simulink model "walkingRobotRL3D"  (R2020b)
settings: Solver=ode23t  StartTime=0.0  StopTime=Tf  RelTol=1e-2  EnableMultiTasking=on
PreLoadFcn:
  | robotParametersRL
undefined symbols (not defined in the file): agent, ankleD_pitch_jointMAX, ankleD_pitch_jointMIN, ankleD_roll_jointMAX, ankleD_roll_jointMIN, ankleI_pitch_jointMAX, ankleI_pitch_jointMIN, ankleI_roll_jointMAX, ankleI_roll_jointMIN, getSampleTime, height_plane, hipD_pitch_jointMAX, hipD_pitch_jointMIN, hipD_roll_jointMAX, hipD_roll_jointMIN, hipI_pitch_jointMAX, hipI_pitch_jointMIN, hipI_roll_jointMAX, hipI_roll_jointMIN, init_angs_L, init_angs_R, init_height, joint_damping, joint_limit_damping, joint_limit_stiffness, joint_stiffness, kneeD_jointMAX, kneeD_jointMIN, kneeI_jointMAX, kneeI_jointMIN, lower_leg_I0, lower_leg_length, lower_leg_mass, lower_leg_x, lower_leg_y, muscle_nominal_length, p10_ankleD_roll, plane_x, plane_y, regulator_type, tau, Tf, torso_height, torso_length, torso_offset_x, torso_offset_z, torso_width, torso_x, torso_y, torso_z, Ts, upper_leg_I0, upper_leg_length, upper_leg_mass, upper_leg_x, upper_leg_y, v10_ankleD_pitch, v10_ankleD_roll, v10_ankleI_pitch, v10_ankleI_roll ... (+41)
libraries: sm_lib x222, simulink x183, nesl_utility x130, walkingRobotUtils x69, rllib x2
(part 18 of 24)

== matlab function walkingRobotRL3D/Walking Robot (Angle based)/Antagonistic PAM Left Leg/kneeI PAM/Proportional Regulator (Muscles 2) ==
  data: V1 input; reg_type input; p1 output
% Author: Eduardo Reyero Ibáñez
% Descrition: In this file it will be implemented the required input for the PAM
function p1  = propReg(V1,reg_type)
%% Proportional pressure regulators VPPM
%Range of Voltage
minVoltage = 0;
maxVoltage = 7.98; % This voltage provide 8 bar of pressure with regulator type 1
p1 = zeros(1,1);
%Select regulartor type
%reg_type = 1; % This will be given by the call of the function
%Limit the voltage
for i=1:length(p1)
if V1(i) >= maxVoltage 
    V1(i) = maxVoltage;
end
end
if reg_type == 1
    f_prop = @(V) 0.99*V+0.1;
    for i=1:length(p1)
    p1(i) = f_prop(V1(i));
    end
elseif reg_type == 2
    f_prop = @(V) 0.594*V+0.06;
    for i=1:length(p1)
    p1(i) = f_prop(V1(i));
    end
else
    f_prop = @(V) 0.198*V+0.02;
    for i=1:length(p1)
    p1(i) = f_prop(V1(i));
    end
end

% figure
% fplot(p1)
% xlim([0 10])
% ylim([0 10])
end

== matlab function walkingRobotRL3D/Walking Robot (Angle based)/Antagonistic PAM Left Leg/kneeI PAM/Spring and damping model/Stimation of spring coefficients ==
  data: P1 input; S1 output; Fload input; dmax1 input; F1 input; dmax1_per input
%Author: Eduardo Reyero
%Description: Calculate spring coefficient

function S1 = calculateSpringCoeff(P1,Fload,dmax1,F1,dmax1_per)
S1=zeros(length(dmax1),1);
%curve1 = @(x,P)  -0.002697-93.8*x+2.917*P+13.05*x^2-0.04264*x*P-0.001793*P^2-0.9395*x^3-0.001597*x^2*P-0.0001142*x*P^2+4.694e-06*P^3+0.03335*x^4+6.106e-06*x^3*P+2.699e-06*x^2*P^2+1.25e-07*x*P^3-5.675e-09*P^4-0.0004611*x^5+9.334e-07*x^4*P-1.221e-08*x^3*P^2-1.463e-09*x^2*P^3-4.929e-11*x*P^4+2.492e-12*P^5;
%F1 = zeros(length(P1),1);
for i=1:length(P1)
 %   F1(i) = curve1(dmax1_per(i),P1(i)); %Should be 0 (or aprox 0)
    S1(i) = (F1(i)-Fload(i))/dmax1(i); 
end
 
 %   S1(i) = 4379.43006090932;
end

== matlab function walkingRobotRL3D/Walking Robot (Angle based)/Antagonistic PAM Left Leg/kneeI PAM/Spring and damping model/Stimation of spring coefficients1 ==
  data: F2 input; P2 input; S2 output; Fload input; dmax2 input; dmax2_per input
%Author: Eduardo Reyero
%Description: Calculate spring coefficient

function S2 = calculateSpringCoeff(F2,P2,Fload,dmax2,dmax2_per)
S2=zeros(length(dmax2),1);
%curve1 = @(x,P)  -0.002697-93.8*x+2.917*P+13.05*x^2-0.04264*x*P-0.001793*P^2-0.9395*x^3-0.001597*x^2*P-0.0001142*x*P^2+4.694e-06*P^3+0.03335*x^4+6.106e-06*x^3*P+2.699e-06*x^2*P^2+1.25e-07*x*P^3-5.675e-09*P^4-0.0004611*x^5+9.334e-07*x^4*P-1.221e-08*x^3*P^2-1.463e-09*x^2*P^3-4.929e-11*x*P^4+2.492e-12*P^5;
%F2 = zeros(length(P2),1);
for i=1:length(P2)
   % F2(i) = curve1(dmax2_per(i),P2(i)); %Should be aprox 0
    S2(i) = (F2(i)-Fload(i))/dmax2(i); 
end
  %  S2(i) = -8268.02654048148;
end

== matlab function walkingRobotRL3D/Walking Robot (Angle based)/Antagonistic PAM Left Leg/kneeI PAM/Spring and damping model/getDeltaXmax/getMaxStroke1 ==
  data: P1 input; x_max1 output
%Author: Eduardo Reyero Ibáñez
%Description: Functions for obtaining the maximun stroke value of a given
%curve F(x). It is reached for the x value which makes F = 0
function x_max1 = getMaxStroke(P1)
x_range = (-3:0.01:29)'; %This range convers the %contraction for all the pressures from 0 to 8 bar
%load('StaticFxPmodel\fxpSurface.mat');

curve1 = @(x,P)  -0.002697-93.8*x+2.917*P+13.05*x^2-0.04264*x*P-0.001793*P^2-0.9395*x^3-0.001597*x^2*P-0.0001142*x*P^2+4.694e-06*P^3+0.03335*x^4+6.106e-06*x^3*P+2.699e-06*x^2*P^2+1.25e-07*x*P^3-5.675e-09*P^4-0.0004611*x^5+9.334e-07*x^4*P-1.221e-08*x^3*P^2-1.463e-09*x^2*P^3-4.929e-11*x*P^4+2.492e-12*P^5;
F_x = zeros(length(x_range),1);
for i=1:length(x_range)
    F_x(i) = curve1(x_range(i),P1);
    if F_x(i)<0
       %We have found the x axis cross
       x_max1 = x_range(i-1);
       break;
   else
        x_max1 = x_range(i); %Will never end here but need to avoid simulink error
    end
end

end

== matlab function walkingRobotRL3D/Walking Robot (Angle based)/Antagonistic PAM Left Leg/kneeI PAM/Spring and damping model/getDeltaXmax1/getMaxStroke1 ==
  data: P2 input; x_max1 output
%Author: Eduardo Reyero Ibáñez
%Description: Functions for obtaining the maximun stroke value of a given
%curve F(x). It is reached for the x value which makes F = 0
function x_max1 = getMaxStroke(P2)
x_range = (-3:0.01:29)'; %This range convers the %contraction for all the pressures from 0 to 8 bar
%load('StaticFxPmodel\fxpSurface.mat');

curve1 = @(x,P)  -0.002697-93.8*x+2.917*P+13.05*x^2-0.04264*x*P-0.001793*P^2-0.9395*x^3-0.001597*x^2*P-0.0001142*x*P^2+4.694e-06*P^3+0.03335*x^4+6.106e-06*x^3*P+2.699e-06*x^2*P^2+1.25e-07*x*P^3-5.675e-09*P^4-0.0004611*x^5+9.334e-07*x^4*P-1.221e-08*x^3*P^2-1.463e-09*x^2*P^3-4.929e-11*x*P^4+2.492e-12*P^5;
F_x = zeros(length(x_range),1);
for i=1:length(x_range)
    F_x(i) = curve1(x_range(i),P2);
    if F_x(i)<0
       %We have found the x axis cross
       x_max1 = x_range(i-1);
       break;
   else
        x_max1 = x_range(i); %Will never end here but need to avoid simulink error
    end
end

end

== matlab function walkingRobotRL3D/Walking Robot (Angle based)/Antagonistic PAM Right Leg/Calculate Torque ==
  data: F1 input; torque output; F2 input; x1 input; x2 input; q output
%Author: Eduardo Reyero
%Description: Calculate torque based on pulley system
function [torque,q] = calculateTorque(F1,F2,x1,x2)
r_pulley = 0.03;
q = 0;
x10_ankleD_roll = 14.06*0.26/100; % In (m)
x20_ankleD_roll = 14.05*0.26/100; % In (m)
torque = (F1(1) - F2(1))*r_pulley;
q =(abs(x1(1)-x10_ankleD_roll)+abs(x2(1)-x20_ankleD_roll))/r_pulley;
if x1 >= x10_ankleD_roll
    q = q;
else
    q = - q;
end
if q > 5*pi/36
    q = 5*pi/36;
end
if q < -7*pi/36
    q = -7*pi/36;
end
end

== matlab function walkingRobotRL3D/Walking Robot1/Dynamic model of antagonistic PAM actuators/Spring//Damping (Muscles 1)/Getxmax1/getMaxStroke3 ==
  data: P1 input; x_max1 output
%Author: Eduardo Reyero Ibáñez
%Description: Functions for obtaining the maximun stroke value of a given
%curve F(x). It is reached for the x value which makes F = 0
function x_max1 = getMaxStroke(P1)
x_range = (-3:0.01:29)'; %This range convers the %contraction for all the pressures from 0 to 8 bar
%load('StaticFxPmodel\fxpSurface.mat');
curve1 = @(x,P)  -0.002697-93.8*x+2.917*P+13.05*x^2-0.04264*x*P-0.001793*P^2-0.9395*x^3-0.001597*x^2*P-0.0001142*x*P^2+4.694e-06*P^3+0.03335*x^4+6.106e-06*x^3*P+2.699e-06*x^2*P^2+1.25e-07*x*P^3-5.675e-09*P^4-0.0004611*x^5+9.334e-07*x^4*P-1.221e-08*x^3*P^2-1.463e-09*x^2*P^3-4.929e-11*x*P^4+2.492e-12*P^5;
F_x = zeros(length(x_range),1);
for i=1:length(x_range)
    F_x(i) = curve1(x_range(i),P1);
    if F_x(i)<0
       %We have found the x axis cross
       x_max1 = x_range(i-1);
       break;
   else
        x_max1 = x_range(i); %Will never end here but need to avoid simulink error
    end
end

end

== matlab function walkingRobotRL3D/Walking Robot (Angle based)/Antagonistic PAM Right Leg/Calculate Torque1 ==
  data: F1 input; torque output; F2 input; x1 input; x2 input; q output
%Author: Eduardo Reyero
%Description: Calculate torque based on pulley system
function [torque,q] = calculateTorque(F1,F2,x1,x2)
r_pulley = 0.03;
q = 0;
x10_ankleD_pitch = 14.06*0.26/100; % In (m)
x20_ankleD_pitch = 14.05*0.26/100; % In (m)
torque = (F1(1) - F2(1))*r_pulley;
q =(abs(x1(1)-x10_ankleD_pitch)+abs(x2(1)-x20_ankleD_pitch))/r_pulley;
if x1 >= x10_ankleD_pitch
    q = q;
else
    q = - q;
end
if q > pi/4
    q = pi/4;
end
if q < -pi/4
    q = -pi/4;
end
end

== matlab function walkingRobotRL3D/Walking Robot (Angle based)/Antagonistic PAM Right Leg/Calculate Torque2 ==
  data: F1 input; torque output; F2 input; x1 input; x2 input; q output
%Author: Eduardo Reyero
%Description: Calculate torque based on pulley system
function [torque,q] = calculateTorque(F1,F2,x1,x2)
r_pulley = 0.05;
q = 0;
x10_kneeD = 0.32*0.26/100; 
x20_kneeD = 28.12*0.26/100;
torque = (F1(1) - F2(1))*r_pulley;
q =(abs(x1(1)-x10_kneeD)+abs(x2(1)-x20_kneeD))/r_pulley; % Knee only moves backwards
if q > pi/2
    q = pi/2;
end
if q < 0
    q = 0;
end
end

== matlab function walkingRobotRL3D/Walking Robot (Angle based)/Antagonistic PAM Right Leg/Calculate Torque3 ==
  data: F1 input; torque output; F2 input; x1 input; x2 input; q output
%Author: Eduardo Reyero
%Description: Calculate torque based on pulley system
function [torque,q] = calculateTorque(F1,F2,x1,x2)
r_pulley = 0.05;
q = 0;
x10_hipD_roll = 14.06*0.26/100; % In (m)
x20_hipD_roll = 14.05*0.26/100; % In (m)
torque = (F1(1) - F2(1))*r_pulley;
q =(abs(x1(1)-x10_hipD_roll)+abs(x2(1)-x20_hipD_roll))/r_pulley;
if x1 >= x10_hipD_roll
    q = q;
else
    q = - q;
end
if q > pi/8
    q = pi/8;
end
if q < -pi/16
    q = -pi/16;
end
end

== matlab function walkingRobotRL3D/Walking Robot (Angle based)/Antagonistic PAM Right Leg/Calculate Torque4 ==
  data: F1 input; torque output; F2 input; x1 input; x2 input; q output
%Author: Eduardo Reyero
%Description: Calculate torque based on pulley system
function [torque,q] = calculateTorque(F1,F2,x1,x2)
r_pulley = 0.05;
q = 0;
x10_hipD_pitch = 14.06*0.26/100; % In (m)
x20_hipD_pitch = 14.05*0.26/100; % In (m)
torque = (F1(1) - F2(1))*r_pulley;
q =(abs(x1(1)-x10_hipD_pitch)+abs(x2(1)-x20_hipD_pitch))/r_pulley;
if x1 >= x10_hipD_pitch
    q = q;
else
    q = - q;
end
if q > pi/4
    q = pi/4;
end
if q < -pi/4
    q = -pi/4;
end
end

== matlab function walkingRobotRL3D/Walking Robot (Angle based)/Antagonistic PAM Left Leg/Calculate Torque ==
  data: F1 input; torque output; F2 input; x1 input; x2 input; q output
%Author: Eduardo Reyero
%Description: Calculate torque based on pulley system
function [torque,q] = calculateTorque(F1,F2,x1,x2)
r_pulley = 0.03;
q = 0;
x10_ankleI_roll = 14.06*0.26/100; % In (m)
x20_ankleI_roll = 14.05*0.26/100; % In (m)
torque = (F1(1) - F2(1))*r_pulley;
q =(abs(x1(1)-x10_ankleI_roll)+abs(x2(1)-x20_ankleI_roll))/r_pulley;
if x1 >= x10_ankleI_roll
    q = q;
else
    q = - q;
end
if q > 7*pi/36
    q = 7*pi/36;
end
if q < -5*pi/36
    q = -5*pi/36;
end
end

== matlab function walkingRobotRL3D/Walking Robot (Angle based)/Antagonistic PAM Left Leg/Calculate Torque1 ==
  data: F1 input; torque output; F2 input; x1 input; x2 input; q output
%Author: Eduardo Reyero
%Description: Calculate torque based on pulley system
function [torque,q] = calculateTorque(F1,F2,x1,x2)
r_pulley = 0.03;
q = 0;
x10_ankleI_pitch = 14.06*0.26/100; % In (m)
x20_ankleI_pitch = 14.05*0.26/100; % In (m)
torque = (F1(1) - F2(1))*r_pulley;
q =(abs(x1(1)-x10_ankleI_pitch)+abs(x2(1)-x20_ankleI_pitch))/r_pulley;
if x1 >= x10_ankleI_pitch
    q = q;
else
    q = - q;
end
if q > pi/4
    q = pi/4;
end
if q < -pi/4
    q = -pi/4;
end
end

== matlab function walkingRobotRL3D/Walking Robot1/Dynamic model of antagonistic PAM actuators/Spring//Damping (Muscles 1)/Getxmax1/getMaxStroke4 ==
  data: P1 input; x_max1 output
%Author: Eduardo Reyero Ibáñez
%Description: Functions for obtaining the maximun stroke value of a given
%curve F(x). It is reached for the x value which makes F = 0
function x_max1 = getMaxStroke(P1)
x_range = (-3:0.01:29)'; %This range convers the %contraction for all the pressures from 0 to 8 bar
%load('StaticFxPmodel\fxpSurface.mat');
curve1 = @(x,P)  -0.002697-93.8*x+2.917*P+13.05*x^2-0.04264*x*P-0.001793*P^2-0.9395*x^3-0.001597*x^2*P-0.0001142*x*P^2+4.694e-06*P^3+0.03335*x^4+6.106e-06*x^3*P+2.699e-06*x^2*P^2+1.25e-07*x*P^3-5.675e-09*P^4-0.0004611*x^5+9.334e-07*x^4*P-1.221e-08*x^3*P^2-1.463e-09*x^2*P^3-4.929e-11*x*P^4+2.492e-12*P^5;
F_x = zeros(length(x_range),1);
for i=1:length(x_range)
    F_x(i) = curve1(x_range(i),P1);
    if F_x(i)<0
       %We have found the x axis cross
       x_max1 = x_range(i-1);
       break;
   else
        x_max1 = x_range(i); %Will never end here but need to avoid simulink error
    end
end

end

== matlab function walkingRobotRL3D/Walking Robot (Angle based)/Antagonistic PAM Left Leg/Calculate Torque2 ==
  data: F1 input; torque output; F2 input; x1 input; x2 input; q output
%Author: Eduardo Reyero
%Description: Calculate torque based on pulley system
function [torque,q] = calculateTorque(F1,F2,x1,x2)
r_pulley = 0.05;
q = 0;
x10_kneeI = 0.32*0.26/100; 
x20_kneeI = 28.12*0.26/100;
torque = (F1(1) - F2(1))*r_pulley;
q =(abs(x1(1)-x10_kneeI)+abs(x2(1)-x20_kneeI))/r_pulley; % Knee only moves backwards
if q > pi/2
    q = pi/2;
end
if q < 0
    q = 0;
end
end

== matlab function walkingRobotRL3D/Walking Robot (Angle based)/Antagonistic PAM Left Leg/Calculate Torque3 ==
  data: F1 input; torque output; F2 input; x1 input; x2 input; q output
%Author: Eduardo Reyero
%Description: Calculate torque based on pulley system
function [torque,q] = calculateTorque(F1,F2,x1,x2)
r_pulley = 0.05;
q = 0;
x10_hipI_roll = 14.06*0.26/100; % In (m)
x20_hipI_roll = 14.05*0.26/100; % In (m)
torque = (F1(1) - F2(1))*r_pulley;
q =(abs(x1(1)-x10_hipI_roll)+abs(x2(1)-x20_hipI_roll))/r_pulley;
if x1 >= x10_hipI_roll
    q = q;
else
    q = - q;
end
if q > pi/16
    q = pi/16;
end
if q < -pi/8
    q = -pi/8;
end
end

== matlab function walkingRobotRL3D/Walking Robot (Angle based)/Antagonistic PAM Left Leg/Calculate Torque4 ==
  data: F1 input; torque output; F2 input; x1 input; x2 input; q output
%Author: Eduardo Reyero
%Description: Calculate torque based on pulley system
function [torque,q] = calculateTorque(F1,F2,x1,x2)
r_pulley = 0.05;
q = 0;
x10_hipI_pitch = 14.06*0.26/100; % In (m)
x20_hipI_pitch = 14.05*0.26/100; % In (m)
torque = (F1(1) - F2(1))*r_pulley;
q =(abs(x1(1)-x10_hipI_pitch)+abs(x2(1)-x20_hipI_pitch))/r_pulley;
if x1 >= x10_hipI_pitch
    q = q;
else
    q = - q;
end
if q > pi/4
    q = pi/4;
end
if q < -pi/4
    q = -pi/4;
end
end

== matlab function walkingRobotRL3D/Walking Robot (Angle based)/Dynamic model of antagonistic PAM actuators/Spring//Damping (Muscles 2)/Getxmax2/Get_delta_xmax1/getDeltaXmax4/getMaxStroke ==
  data: P2 input; x_max2 output
%Author: Eduardo Reyero Ibáñez
%Description: Functions for obtaining the maximun stroke value of a given
%curve F(x). It is reached for the x value which makes F = 0
function x_max2 = getMaxStroke(P2)
x_range = (-3:0.01:29)'; %This range convers the %contraction for all the pressures from 0 to 8 bar
%load('StaticFxPmodel\fxpSurface.mat');
curve1 = @(x,P)  -0.002697-93.8*x+2.917*P+13.05*x^2-0.04264*x*P-0.001793*P^2-0.9395*x^3-0.001597*x^2*P-0.0001142*x*P^2+4.694e-06*P^3+0.03335*x^4+6.106e-06*x^3*P+2.699e-06*x^2*P^2+1.25e-07*x*P^3-5.675e-09*P^4-0.0004611*x^5+9.334e-07*x^4*P-1.221e-08*x^3*P^2-1.463e-09*x^2*P^3-4.929e-11*x*P^4+2.492e-12*P^5;
F_x = zeros(length(x_range),1);
for i=1:length(x_range)
    F_x(i) = curve1(x_range(i),P2);
    if F_x(i)<0
       %We have found the x axis cross
       x_max2 = x_range(i-1);
       break;
   else
        x_max2 = x_range(i); %Will never end here but need to avoid simulink error
    end
end

end

== matlab function walkingRobotRL3D/Walking Robot (Angle based)/Dynamic model of antagonistic PAM actuators/Spring//Damping (Muscles 2)/Getxmax2/Get_delta_xmax1/getDeltaXmax5/MATLAB Function ==
  data: x input; savex output; xant input; save input
function savex = fcn(x,xant,save)
dif = x-xant;
if dif ~=0
    savex = xant;
else
    savex = save; %Will be the previous
end
end

== matlab function walkingRobotRL3D/Walking Robot (Angle based)/Dynamic model of antagonistic PAM actuators/Spring//Damping (Muscles 2)/Getxmax2/Get_delta_xmax1/getDeltaXmax5/getMaxStroke ==
  data: P2 input; x_max2 output
%Author: Eduardo Reyero Ibáñez
%Description: Functions for obtaining the maximun stroke value of a given
%curve F(x). It is reached for the x value which makes F = 0
function x_max2 = getMaxStroke(P2)
x_range = (-3:0.01:29)'; %This range convers the %contraction for all the pressures from 0 to 8 bar
%load('StaticFxPmodel\fxpSurface.mat');
curve1 = @(x,P)  -0.002697-93.8*x+2.917*P+13.05*x^2-0.04264*x*P-0.001793*P^2-0.9395*x^3-0.001597*x^2*P-0.0001142*x*P^2+4.694e-06*P^3+0.03335*x^4+6.106e-06*x^3*P+2.699e-06*x^2*P^2+1.25e-07*x*P^3-5.675e-09*P^4-0.0004611*x^5+9.334e-07*x^4*P-1.221e-08*x^3*P^2-1.463e-09*x^2*P^3-4.929e-11*x*P^4+2.492e-12*P^5;
F_x = zeros(length(x_range),1);
for i=1:length(x_range)
    F_x(i) = curve1(x_range(i),P2);
    if F_x(i)<0
       %We have found the x axis cross
       x_max2 = x_range(i-1);
       break;
   else
        x_max2 = x_range(i); %Will never end here but need to avoid simulink error
    end
end

end

== matlab function walkingRobotRL3D/Walking Robot (Angle based)/Dynamic model of antagonistic PAM actuators/Spring//Damping (Muscles 2)/Getxmax2/Get_delta_xmax1/getDeltaXmax6/MATLAB Function ==
  data: x input; savex output; xant input; save input
function savex = fcn(x,xant,save)
dif = x-xant;
if dif ~=0
    savex = xant;
else
    savex = save; %Will be the previous
end
end

== matlab function walkingRobotRL3D/Walking Robot (Angle based)/Dynamic model of antagonistic PAM actuators/Spring//Damping (Muscles 2)/Getxmax2/Get_delta_xmax1/getDeltaXmax6/getMaxStroke ==
  data: P2 input; x_max2 output
%Author: Eduardo Reyero Ibáñez
%Description: Functions for obtaining the maximun stroke value of a given
%curve F(x). It is reached for the x value which makes F = 0
function x_max2 = getMaxStroke(P2)
x_range = (-3:0.01:29)'; %This range convers the %contraction for all the pressures from 0 to 8 bar
%load('StaticFxPmodel\fxpSurface.mat');
curve1 = @(x,P)  -0.002697-93.8*x+2.917*P+13.05*x^2-0.04264*x*P-0.001793*P^2-0.9395*x^3-0.001597*x^2*P-0.0001142*x*P^2+4.694e-06*P^3+0.03335*x^4+6.106e-06*x^3*P+2.699e-06*x^2*P^2+1.25e-07*x*P^3-5.675e-09*P^4-0.0004611*x^5+9.334e-07*x^4*P-1.221e-08*x^3*P^2-1.463e-09*x^2*P^3-4.929e-11*x*P^4+2.492e-12*P^5;
F_x = zeros(length(x_range),1);
for i=1:length(x_range)
    F_x(i) = curve1(x_range(i),P2);
    if F_x(i)<0
       %We have found the x axis cross
       x_max2 = x_range(i-1);
       break;
   else
        x_max2 = x_range(i); %Will never end here but need to avoid simulink error
    end
end

end

== matlab function walkingRobotRL3D/Walking Robot1/Dynamic model of antagonistic PAM actuators/Spring//Damping (Muscles 1)/Getxmax1/getMaxStroke5 ==
  data: P1 input; x_max1 output
%Author: Eduardo Reyero Ibáñez
%Description: Functions for obtaining the maximun stroke value of a given
%curve F(x). It is reached for the x value which makes F = 0
function x_max1 = getMaxStroke(P1)
x_range = (-3:0.01:29)'; %This range convers the %contraction for all the pressures from 0 to 8 bar
%load('StaticFxPmodel\fxpSurface.mat');
curve1 = @(x,P)  -0.002697-93.8*x+2.917*P+13.05*x^2-0.04264*x*P-0.001793*P^2-0.9395*x^3-0.001597*x^2*P-0.0001142*x*P^2+4.694e-06*P^3+0.03335*x^4+6.106e-06*x^3*P+2.699e-06*x^2*P^2+1.25e-07*x*P^3-5.675e-09*P^4-0.0004611*x^5+9.334e-07*x^4*P-1.221e-08*x^3*P^2-1.463e-09*x^2*P^3-4.929e-11*x*P^4+2.492e-12*P^5;
F_x = zeros(length(x_range),1);
for i=1:length(x_range)
    F_x(i) = curve1(x_range(i),P1);
    if F_x(i)<0
       %We have found the x axis cross
       x_max1 = x_range(i-1);
       break;
   else
        x_max1 = x_range(i); %Will never end here but need to avoid simulink error
    end
end

end

== matlab function walkingRobotRL3D/Walking Robot (Angle based)/Dynamic model of antagonistic PAM actuators/Spring//Damping (Muscles 2)/Getxmax2/Get_delta_xmax1/getDeltaXmax7/MATLAB Function ==
  data: x input; savex output; xant input; save input
function savex = fcn(x,xant,save)
dif = x-xant;
if dif ~=0
    savex = xant;
else
    savex = save; %Will be the previous
end
end

== matlab function walkingRobotRL3D/Walking Robot (Angle based)/Dynamic model of antagonistic PAM actuators/Spring//Damping (Muscles 2)/Getxmax2/Get_delta_xmax1/getDeltaXmax7/getMaxStroke ==
  data: P2 input; x_max2 output
%Author: Eduardo Reyero Ibáñez
%Description: Functions for obtaining the maximun stroke value of a given
%curve F(x). It is reached for the x value which makes F = 0
function x_max2 = getMaxStroke(P2)
x_range = (-3:0.01:29)'; %This range convers the %contraction for all the pressures from 0 to 8 bar
%load('StaticFxPmodel\fxpSurface.mat');
curve1 = @(x,P)  -0.002697-93.8*x+2.917*P+13.05*x^2-0.04264*x*P-0.001793*P^2-0.9395*x^3-0.001597*x^2*P-0.0001142*x*P^2+4.694e-06*P^3+0.03335*x^4+6.106e-06*x^3*P+2.699e-06*x^2*P^2+1.25e-07*x*P^3-5.675e-09*P^4-0.0004611*x^5+9.334e-07*x^4*P-1.221e-08*x^3*P^2-1.463e-09*x^2*P^3-4.929e-11*x*P^4+2.492e-12*P^5;
F_x = zeros(length(x_range),1);
for i=1:length(x_range)
    F_x(i) = curve1(x_range(i),P2);
    if F_x(i)<0
       %We have found the x axis cross
       x_max2 = x_range(i-1);
       break;
   else
        x_max2 = x_range(i); %Will never end here but need to avoid simulink error
    end
end

end

== matlab function walkingRobotRL3D/Walking Robot (Angle based)/Dynamic model of antagonistic PAM actuators/Spring//Damping (Muscles 2)/Getxmax2/Get_delta_xmax1/getDeltaXmax8/MATLAB Function ==
  data: x input; savex output; xant input; save input
function savex = fcn(x,xant,save)
dif = x-xant;
if dif ~=0
    savex = xant;
else
    savex = save; %Will be the previous
end
end

== matlab function walkingRobotRL3D/Walking Robot (Angle based)/Dynamic model of antagonistic PAM actuators/Spring//Damping (Muscles 2)/Getxmax2/Get_delta_xmax1/getDeltaXmax8/getMaxStroke ==
  data: P2 input; x_max2 output
%Author: Eduardo Reyero Ibáñez
%Description: Functions for obtaining the maximun stroke value of a given
%curve F(x). It is reached for the x value which makes F = 0
function x_max2 = getMaxStroke(P2)
x_range = (-3:0.01:29)'; %This range convers the %contraction for all the pressures from 0 to 8 bar
%load('StaticFxPmodel\fxpSurface.mat');
curve1 = @(x,P)  -0.002697-93.8*x+2.917*P+13.05*x^2-0.04264*x*P-0.001793*P^2-0.9395*x^3-0.001597*x^2*P-0.0001142*x*P^2+4.694e-06*P^3+0.03335*x^4+6.106e-06*x^3*P+2.699e-06*x^2*P^2+1.25e-07*x*P^3-5.675e-09*P^4-0.0004611*x^5+9.334e-07*x^4*P-1.221e-08*x^3*P^2-1.463e-09*x^2*P^3-4.929e-11*x*P^4+2.492e-12*P^5;
F_x = zeros(length(x_range),1);
for i=1:length(x_range)
    F_x(i) = curve1(x_range(i),P2);
    if F_x(i)<0
       %We have found the x axis cross
       x_max2 = x_range(i-1);
       break;
   else
        x_max2 = x_range(i); %Will never end here but need to avoid simulink error
    end
end

end

== matlab function walkingRobotRL3D/Walking Robot (Angle based)/Dynamic model of antagonistic PAM actuators/Spring//Damping (Muscles 2)/Getxmax2/Get_delta_xmax1/getDeltaXmax9/MATLAB Function ==
  data: x input; savex output; xant input; save input
function savex = fcn(x,xant,save)
dif = x-xant;
if dif ~=0
    savex = xant;
else
    savex = save; %Will be the previous
end
end

== matlab function walkingRobotRL3D/Walking Robot (Angle based)/Dynamic model of antagonistic PAM actuators/Spring//Damping (Muscles 2)/Getxmax2/Get_delta_xmax1/getDeltaXmax9/getMaxStroke ==
  data: P2 input; x_max2 output
%Author: Eduardo Reyero Ibáñez
%Description: Functions for obtaining the maximun stroke value of a given
%curve F(x). It is reached for the x value which makes F = 0
function x_max2 = getMaxStroke(P2)
x_range = (-3:0.01:29)'; %This range convers the %contraction for all the pressures from 0 to 8 bar
%load('StaticFxPmodel\fxpSurface.mat');
curve1 = @(x,P)  -0.002697-93.8*x+2.917*P+13.05*x^2-0.04264*x*P-0.001793*P^2-0.9395*x^3-0.001597*x^2*P-0.0001142*x*P^2+4.694e-06*P^3+0.03335*x^4+6.106e-06*x^3*P+2.699e-06*x^2*P^2+1.25e-07*x*P^3-5.675e-09*P^4-0.0004611*x^5+9.334e-07*x^4*P-1.221e-08*x^3*P^2-1.463e-09*x^2*P^3-4.929e-11*x*P^4+2.492e-12*P^5;
F_x = zeros(length(x_range),1);
for i=1:length(x_range)
    F_x(i) = curve1(x_range(i),P2);
    if F_x(i)<0
       %We have found the x axis cross
       x_max2 = x_range(i-1);
       break;
   else
        x_max2 = x_range(i); %Will never end here but need to avoid simulink error
    end
end

end

== matlab function walkingRobotRL3D/Walking Robot (Angle based)/Dynamic model of antagonistic PAM actuators/Spring//Damping (Muscles 2)/MATLAB Function ==
  data: P1 input; S2 output; P2 input; delta_xmax_muscles2 input; delta_xmax_muscles1_per input; delta_xmax_muscles2_per input
%Author: Eduardo Reyero
%Description: Calculate spring coefficient

function S2 = calculateSpringCoeff2(P1,P2,delta_xmax_muscles2,delta_xmax_muscles1_per,delta_xmax_muscles2_per)
S2=zeros(length(delta_xmax_muscles2),1);
curve1 = @(x,P)  -0.002697-93.8*x+2.917*P+13.05*x^2-0.04264*x*P-0.001793*P^2-0.9395*x^3-0.001597*x^2*P-0.0001142*x*P^2+4.694e-06*P^3+0.03335*x^4+6.106e-06*x^3*P+2.699e-06*x^2*P^2+1.25e-07*x*P^3-5.675e-09*P^4-0.0004611*x^5+9.334e-07*x^4*P-1.221e-08*x^3*P^2-1.463e-09*x^2*P^3-4.929e-11*x*P^4+2.492e-12*P^5;
F1 = zeros(length(P1),1);
F2 = zeros(length(P1),1);
for i = 1:length(P2)
   F1(i) = curve1(delta_xmax_muscles1_per(i),P1(i));
   F2(i) = curve1(delta_xmax_muscles2_per(i),P2(i));
  S2(i) = (F2(i)-F1(i))/delta_xmax_muscles2(i);
  %S2(i) = F2(i)-F1(i)/(delta_xmax_muscles2_per(i)*0.26/100);
  
%    if S2(i)> 1e+05 || S2(i)< -1e+05
%        S2(i) = 0.1;
%    end
%    if S2(i)<0
%    S2(i) = -S2(i); 
%    end
end

end

== matlab function walkingRobotRL3D/Action+CI1/MATLAB Function ==
  data: x1 input; v1 output; v2 output
function [v1,v2]=ankleD_action(x1)
v1_values = [1.6809 1.72]';
v2_values = [1.6807 1.64]';
v1 = v1_values(1);
v2 = v2_values(1);
if  x1(1)>=14.05 
    v1 = v1_values(2);
    v2 = v2_values(2);
end
  
end

== matlab function walkingRobotRL3D/Walking Robot33/DYNAMIC MODEL OF PAM FOR LEFT LEG/Dynamic Model Antagonisitic PAM1/F(x,P) mode (Muscles 1) ==
  data: P1 input; F1 output; x_muscle1 input
%Author: Eduardo Reyero Ibáñez
%Note: F(x) curves for different pressures are limited by recommended
%limitation of 20% in contraction percentage for the used PAM actuator
%(L = 260mm D=20mm)
function F1 = FxPmodel(P1,x_muscle1)
%Input: P comming from proporcional controller  is in bar. Its 6x1 vector
% x_muscle (in % contraction)
%Output:F according to P input and and x value of half of the maximun
%permissible stroke
%Importing 2 variable F(x,P) model
curve = @(x,P)  -0.002697-93.8*x+2.917*P+13.05*x^2-0.04264*x*P-0.001793*P^2-0.9395*x^3-0.001597*x^2*P-0.0001142*x*P^2+4.694e-06*P^3+0.03335*x^4+6.106e-06*x^3*P+2.699e-06*x^2*P^2+1.25e-07*x*P^3-5.675e-09*P^4-0.0004611*x^5+9.334e-07*x^4*P-1.221e-08*x^3*P^2-1.463e-09*x^2*P^3-4.929e-11*x*P^4+2.492e-12*P^5;
%Defining F and x vectors for the 6 actuators
F1 = zeros(length(P1),1); %6x1
x1 = zeros(length(P1),1); %6x1
% Transform P from bar to Kpa
P1 = 100*P1;

for i=1:length(P1)
% Obtaining the stroke
x1(i) = x_muscle1(i); 
% Obtaining the applied force
F1(i) = curve(x1(i),P1(i)); 
if F1(i)<0
    F1(i) = 0;
end
end
end

== matlab function walkingRobotRL3D/Walking Robot1/Dynamic model of antagonistic PAM actuators/Spring//Damping (Muscles 2)/Getxmax2/getMaxStroke7 ==
  data: P2 input; x_max2 output
%Author: Eduardo Reyero Ibáñez
%Description: Functions for obtaining the maximun stroke value of a given
%curve F(x). It is reached for the x value which makes F = 0
function x_max2 = getMaxStroke(P2)
x_range = (-3:0.01:29)'; %This range convers the %contraction for all the pressures from 0 to 8 bar
%load('StaticFxPmodel\fxpSurface.mat');
curve1 = @(x,P)  -0.002697-93.8*x+2.917*P+13.05*x^2-0.04264*x*P-0.001793*P^2-0.9395*x^3-0.001597*x^2*P-0.0001142*x*P^2+4.694e-06*P^3+0.03335*x^4+6.106e-06*x^3*P+2.699e-06*x^2*P^2+1.25e-07*x*P^3-5.675e-09*P^4-0.0004611*x^5+9.334e-07*x^4*P-1.221e-08*x^3*P^2-1.463e-09*x^2*P^3-4.929e-11*x*P^4+2.492e-12*P^5;
F_x = zeros(length(x_range),1);
for i=1:length(x_range)
    F_x(i) = curve1(x_range(i),P2);
    if F_x(i)<0
       %We have found the x axis cross
       x_max2 = x_range(i-1);
       break;
   else
        x_max2 = x_range(i); %Will never end here but need to avoid simulink error
    end
end

end

== matlab function walkingRobotRL3D/Walking Robot33/DYNAMIC MODEL OF PAM FOR LEFT LEG/Dynamic Model Antagonisitic PAM1/F(x,P) mode (Muscles 1)1 ==
  data: P2 input; F2 output; x_muscle2 input
%Author: Eduardo Reyero Ibáñez
%Note: F(x) curves for different pressures are limited by recommended
%limitation of 20% in contraction percentage for the used PAM actuator
%(L = 260mm D=20mm)
function F2 = FxPmodel(P2,x_muscle2)
%Input: P comming from proporcional controller  is in bar. Its 6x1 vector
% x_muscle (in % contraction)
%Output:F according to P input and and x value of half of the maximun
%permissible stroke
%Importing 2 variable F(x,P) model
curve = @(x,P)  -0.002697-93.8*x+2.917*P+13.05*x^2-0.04264*x*P-0.001793*P^2-0.9395*x^3-0.001597*x^2*P-0.0001142*x*P^2+4.694e-06*P^3+0.03335*x^4+6.106e-06*x^3*P+2.699e-06*x^2*P^2+1.25e-07*x*P^3-5.675e-09*P^4-0.0004611*x^5+9.334e-07*x^4*P-1.221e-08*x^3*P^2-1.463e-09*x^2*P^3-4.929e-11*x*P^4+2.492e-12*P^5;
%Defining F and x vectors for the 6 actuators
F2 = zeros(length(P2),1); %6x1
x2 = zeros(length(P2),1); %6x1
% Transform P from bar to Kpa
P2 = 100*P2;

for i=1:length(P2)
% Obtaining the stroke
x2(i) = x_muscle2(i); 
% Obtaining the applied force
F2(i) = curve(x2(i),P2(i));
if F2(i)<0
    F2(i) = 0;
end
end
end

== matlab function walkingRobotRL3D/Walking Robot33/DYNAMIC MODEL OF PAM FOR LEFT LEG/Dynamic Model Antagonisitic PAM1/Proportional Regulator (Muscles 1) ==
  data: V1 input; reg_type input; p1 output
% Author: Eduardo Reyero Ibáñez
% Descrition: In this file it will be implemented the required input for the PAM
function p1  = propReg(V1,reg_type)
%% Proportional pressure regulators VPPM
%Range of Voltage
minVoltage = 0;
maxVoltage = 7.98; % This voltage provide 8 bar of pressure with regulator type 1
p1 = zeros(1,1);
%Select regulartor type
%reg_type = 1; % This will be given by the call of the function
%Limit the voltage
for i=1:length(p1)
if V1(i) >= maxVoltage 
    V1(i) = maxVoltage;
end
end
if reg_type == 1
    f_prop = @(V) 0.99*V+0.1;
    for i=1:length(p1)
    p1(i) = f_prop(V1(i));
    end
elseif reg_type == 2
    f_prop = @(V) 0.594*V+0.06;
    for i=1:length(p1)
    p1(i) = f_prop(V1(i));
    end
else
    f_prop = @(V) 0.198*V+0.02;
    for i=1:length(p1)
    p1(i) = f_prop(V1(i));
    end
end

% figure
% fplot(p1)
% xlim([0 10])
% ylim([0 10])
end

== matlab function walkingRobotRL3D/Walking Robot33/DYNAMIC MODEL OF PAM FOR LEFT LEG/Dynamic Model Antagonisitic PAM1/Proportional Regulator (Muscles 2) ==
  data: V1 input; reg_type input; p1 output
% Author: Eduardo Reyero Ibáñez
% Descrition: In this file it will be implemented the required input for the PAM
function p1  = propReg(V1,reg_type)
%% Proportional pressure regulators VPPM
%Range of Voltage
minVoltage = 0;
maxVoltage = 7.98; % This voltage provide 8 bar of pressure with regulator type 1
p1 = zeros(1,1);
%Select regulartor type
%reg_type = 1; % This will be given by the call of the function
%Limit the voltage
for i=1:length(p1)
if V1(i) >= maxVoltage 
    V1(i) = maxVoltage;
end
end
if reg_type == 1
    f_prop = @(V) 0.99*V+0.1;
    for i=1:length(p1)
    p1(i) = f_prop(V1(i));
    end
elseif reg_type == 2
    f_prop = @(V) 0.594*V+0.06;
    for i=1:length(p1)
    p1(i) = f_prop(V1(i));
    end
else
    f_prop = @(V) 0.198*V+0.02;
    for i=1:length(p1)
    p1(i) = f_prop(V1(i));
    end
end

% figure
% fplot(p1)
% xlim([0 10])
% ylim([0 10])
end

== matlab function walkingRobotRL3D/Walking Robot33/DYNAMIC MODEL OF PAM FOR LEFT LEG/Dynamic Model Antagonisitic PAM1/Spring and damping model/S(P),D(P) ==
  data: P1 input; S1 output; P2 input; D1 output; S2 output; D2 output
function [S1,D1,S2,D2] = getSpringDampingCoeff(P1,P2)
tau = 0.6;
% Spring and damping coeff for muscle 1
if P1>=0 && P1<=1
    S1 = 400;
    D1 = tau*S1;
elseif P1>1 && P1<=2
    S1 = 500;
    D1 = tau*S1;
elseif P1>2 && P1<=3
    S1 = 1100;
    D1 = tau*S1;
elseif P1>3 && P1<=4
    S1 = 1500;
    D1 = tau*S1;
elseif P1>4 && P1<=5
    S1 = 2000;
    D1 = tau*S1;
elseif P1>5 && P1<=6
    S1 = 2900;
    D1 = tau*S1;
elseif P1>6 && P1<=7
    S1 = 3800;
    D1 = tau*S1;
elseif P1>7 && P1<=8.5
    S1 = 5000;
    D1 = tau*S1;
else %Never will enter here
    S1 = 800;
    D1 = tau*S1;  
end

% Spring and damping coeff for muscle 1
if P2>=0 && P2<=1
    S2 = 400;
    D2 = tau*S2;
elseif P2>1 && P2<=2
    S2 = 500;
    D2 = tau*S2;
elseif P2>2 && P2<=3
    S2 = 1100;
    D2 = tau*S2;
elseif P2>3 && P2<=4
    S2 = 1500;
    D2 = tau*S2;
elseif P2>4 && P2<=5
    S2 = 2000;
    D2 = tau*S2;
elseif P2>5 && P2<=6
    S2 = 2900;
    D2 = tau*S2;
elseif P2>6 && P2<=7
    S2 = 3800;
    D2 = tau*S2;
elseif P2>7 && P2<=8.5
    S2 = 5000;
    D2 = tau*S2;
else %Never will enter here
    S2 = 800;
    D2 = tau*S2;  
end

end

== matlab function walkingRobotRL3D/Walking Robot33/DYNAMIC MODEL OF PAM FOR LEFT LEG/Dynamic Model Antagonisitic PAM2/F(x,P) mode (Muscles 1) ==
  data: P1 input; F1 output; x_muscle1 input
%Author: Eduardo Reyero Ibáñez
%Note: F(x) curves for different pressures are limited by recommended
%limitation of 20% in contraction percentage for the used PAM actuator
%(L = 260mm D=20mm)
function F1 = FxPmodel(P1,x_muscle1)
%Input: P comming from proporcional controller  is in bar. Its 6x1 vector
% x_muscle (in % contraction)
%Output:F according to P input and and x value of half of the maximun
%permissible stroke
%Importing 2 variable F(x,P) model
curve = @(x,P)  -0.002697-93.8*x+2.917*P+13.05*x^2-0.04264*x*P-0.001793*P^2-0.9395*x^3-0.001597*x^2*P-0.0001142*x*P^2+4.694e-06*P^3+0.03335*x^4+6.106e-06*x^3*P+2.699e-06*x^2*P^2+1.25e-07*x*P^3-5.675e-09*P^4-0.0004611*x^5+9.334e-07*x^4*P-1.221e-08*x^3*P^2-1.463e-09*x^2*P^3-4.929e-11*x*P^4+2.492e-12*P^5;
%Defining F and x vectors for the 6 actuators
F1 = zeros(length(P1),1); %6x1
x1 = zeros(length(P1),1); %6x1
% Transform P from bar to Kpa
P1 = 100*P1;

for i=1:length(P1)
% Obtaining the stroke
x1(i) = x_muscle1(i); 
% Obtaining the applied force
F1(i) = curve(x1(i),P1(i)); 
if F1(i)<0
    F1(i) = 0;
end
end
end

== matlab function walkingRobotRL3D/Walking Robot33/DYNAMIC MODEL OF PAM FOR LEFT LEG/Dynamic Model Antagonisitic PAM2/F(x,P) mode (Muscles 1)1 ==
  data: P2 input; F2 output; x_muscle2 input
%Author: Eduardo Reyero Ibáñez
%Note: F(x) curves for different pressures are limited by recommended
%limitation of 20% in contraction percentage for the used PAM actuator
%(L = 260mm D=20mm)
function F2 = FxPmodel(P2,x_muscle2)
%Input: P comming from proporcional controller  is in bar. Its 6x1 vector
% x_muscle (in % contraction)
%Output:F according to P input and and x value of half of the maximun
%permissible stroke
%Importing 2 variable F(x,P) model
curve = @(x,P)  -0.002697-93.8*x+2.917*P+13.05*x^2-0.04264*x*P-0.001793*P^2-0.9395*x^3-0.001597*x^2*P-0.0001142*x*P^2+4.694e-06*P^3+0.03335*x^4+6.106e-06*x^3*P+2.699e-06*x^2*P^2+1.25e-07*x*P^3-5.675e-09*P^4-0.0004611*x^5+9.334e-07*x^4*P-1.221e-08*x^3*P^2-1.463e-09*x^2*P^3-4.929e-11*x*P^4+2.492e-12*P^5;
%Defining F and x vectors for the 6 actuators
F2 = zeros(length(P2),1); %6x1
x2 = zeros(length(P2),1); %6x1
% Transform P from bar to Kpa
P2 = 100*P2;

for i=1:length(P2)
% Obtaining the stroke
x2(i) = x_muscle2(i); 
% Obtaining the applied force
F2(i) = curve(x2(i),P2(i));
if F2(i)<0
    F2(i) = 0;
end
end
end

== matlab function walkingRobotRL3D/Walking Robot33/DYNAMIC MODEL OF PAM FOR LEFT LEG/Dynamic Model Antagonisitic PAM2/Proportional Regulator (Muscles 1) ==
  data: V1 input; reg_type input; p1 output
% Author: Eduardo Reyero Ibáñez
% Descrition: In this file it will be implemented the required input for the PAM
function p1  = propReg(V1,reg_type)
%% Proportional pressure regulators VPPM
%Range of Voltage
minVoltage = 0;
maxVoltage = 7.98; % This voltage provide 8 bar of pressure with regulator type 1
p1 = zeros(1,1);
%Select regulartor type
%reg_type = 1; % This will be given by the call of the function
%Limit the voltage
for i=1:length(p1)
if V1(i) >= maxVoltage 
    V1(i) = maxVoltage;
end
end
if reg_type == 1
    f_prop = @(V) 0.99*V+0.1;
    for i=1:length(p1)
    p1(i) = f_prop(V1(i));
    end
elseif reg_type == 2
    f_prop = @(V) 0.594*V+0.06;
    for i=1:length(p1)
    p1(i) = f_prop(V1(i));
    end
else
    f_prop = @(V) 0.198*V+0.02;
    for i=1:length(p1)
    p1(i) = f_prop(V1(i));
    end
end

% figure
% fplot(p1)
% xlim([0 10])
% ylim([0 10])
end

== matlab function walkingRobotRL3D/Walking Robot33/DYNAMIC MODEL OF PAM FOR LEFT LEG/Dynamic Model Antagonisitic PAM2/Proportional Regulator (Muscles 2) ==
  data: V1 input; reg_type input; p1 output
% Author: Eduardo Reyero Ibáñez
% Descrition: In this file it will be implemented the required input for the PAM
function p1  = propReg(V1,reg_type)
%% Proportional pressure regulators VPPM
%Range of Voltage
minVoltage = 0;
maxVoltage = 7.98; % This voltage provide 8 bar of pressure with regulator type 1
p1 = zeros(1,1);
%Select regulartor type
%reg_type = 1; % This will be given by the call of the function
%Limit the voltage
for i=1:length(p1)
if V1(i) >= maxVoltage 
    V1(i) = maxVoltage;
end
end
if reg_type == 1
    f_prop = @(V) 0.99*V+0.1;
    for i=1:length(p1)
    p1(i) = f_prop(V1(i));
    end
elseif reg_type == 2
    f_prop = @(V) 0.594*V+0.06;
    for i=1:length(p1)
    p1(i) = f_prop(V1(i));
    end
else
    f_prop = @(V) 0.198*V+0.02;
    for i=1:length(p1)
    p1(i) = f_prop(V1(i));
    end
end

% figure
% fplot(p1)
% xlim([0 10])
% ylim([0 10])
end

== matlab function walkingRobotRL3D/Walking Robot1/Dynamic model of antagonistic PAM actuators/Spring//Damping (Muscles 2)/Getxmax2/getMaxStroke ==
  data: P2 input; x_max2 output
%Author: Eduardo Reyero Ibáñez
%Description: Functions for obtaining the maximun stroke value of a given
%curve F(x). It is reached for the x value which makes F = 0
function x_max2 = getMaxStroke(P2)
x_range = (-3:0.01:29)'; %This range convers the %contraction for all the pressures from 0 to 8 bar
%load('StaticFxPmodel\fxpSurface.mat');
curve1 = @(x,P)  -0.002697-93.8*x+2.917*P+13.05*x^2-0.04264*x*P-0.001793*P^2-0.9395*x^3-0.001597*x^2*P-0.0001142*x*P^2+4.694e-06*P^3+0.03335*x^4+6.106e-06*x^3*P+2.699e-06*x^2*P^2+1.25e-07*x*P^3-5.675e-09*P^4-0.0004611*x^5+9.334e-07*x^4*P-1.221e-08*x^3*P^2-1.463e-09*x^2*P^3-4.929e-11*x*P^4+2.492e-12*P^5;
F_x = zeros(length(x_range),1);
for i=1:length(x_range)
    F_x(i) = curve1(x_range(i),P2);
    if F_x(i)<0
       %We have found the x axis cross
       x_max2 = x_range(i-1);
       break;
   else
        x_max2 = x_range(i); %Will never end here but need to avoid simulink error
    end
end

end

== matlab function walkingRobotRL3D/Action+CI33/MATLAB Function ==
  data: x1 input; v1 output; v2 output
function [v1,v2]=ankleD_action(x1)
v1_values = [1.6809 1.72]';
v2_values = [1.6807 1.64]';
v1 = v1_values(1);
v2 = v2_values(1);
if  x1(1)>=14.05 
    v1 = v1_values(2);
    v2 = v2_values(2);
end
  
end

== matlab function walkingRobotRL3D/mapActions33 ==
  data: value input; output output
function output = mapfun(value)
%narginchk(20,20)
%nargoutchk(0,20)
fromLow = -1;
fromHigh= 1;
toLow= 1.4;
toHigh= 3;
output = (value - fromLow) .* (toHigh - toLow) ./ (fromHigh - fromLow) + toLow;
end

== matlab function walkingRobotRL3D/Walking Robot/DYNAMIC MODEL OF PAM FOR LEFT LEG/Dynamic Model Antagonisitic PAM1/F(x,P) mode (Muscles 1) ==
  data: P1 input; F1 output; x_muscle1 input
%Author: Eduardo Reyero Ibáñez
%Note: F(x) curves for different pressures are limited by recommended
%limitation of 20% in contraction percentage for the used PAM actuator
%(L = 260mm D=20mm)
function F1 = FxPmodel(P1,x_muscle1)
%Input: P comming from proporcional controller  is in bar. Its 6x1 vector
% x_muscle (in % contraction)
%Output:F according to P input and and x value of half of the maximun
%permissible stroke
%Importing 2 variable F(x,P) model
curve = @(x,P)  -0.002697-93.8*x+2.917*P+13.05*x^2-0.04264*x*P-0.001793*P^2-0.9395*x^3-0.001597*x^2*P-0.0001142*x*P^2+4.694e-06*P^3+0.03335*x^4+6.106e-06*x^3*P+2.699e-06*x^2*P^2+1.25e-07*x*P^3-5.675e-09*P^4-0.0004611*x^5+9.334e-07*x^4*P-1.221e-08*x^3*P^2-1.463e-09*x^2*P^3-4.929e-11*x*P^4+2.492e-12*P^5;
%Defining F and x vectors for the 6 actuators
F1 = zeros(length(P1),1); %6x1
x1 = zeros(length(P1),1); %6x1
% Transform P from bar to Kpa
P1 = 100*P1;

for i=1:length(P1)
% Obtaining the stroke
x1(i) = x_muscle1(i); 
% Obtaining the applied force
F1(i) = curve(x1(i),P1(i)); 
if F1(i)<0
    F1(i) = 0;
end
end
end

== matlab function walkingRobotRL3D/Walking Robot/DYNAMIC MODEL OF PAM FOR LEFT LEG/Dynamic Model Antagonisitic PAM1/F(x,P) mode (Muscles 1)1 ==
  data: P2 input; F2 output; x_muscle2 input
%Author: Eduardo Reyero Ibáñez
%Note: F(x) curves for different pressures are limited by recommended
%limitation of 20% in contraction percentage for the used PAM actuator
%(L = 260mm D=20mm)
function F2 = FxPmodel(P2,x_muscle2)
%Input: P comming from proporcional controller  is in bar. Its 6x1 vector
% x_muscle (in % contraction)
%Output:F according to P input and and x value of half of the maximun
%permissible stroke
%Importing 2 variable F(x,P) model
curve = @(x,P)  -0.002697-93.8*x+2.917*P+13.05*x^2-0.04264*x*P-0.001793*P^2-0.9395*x^3-0.001597*x^2*P-0.0001142*x*P^2+4.694e-06*P^3+0.03335*x^4+6.106e-06*x^3*P+2.699e-06*x^2*P^2+1.25e-07*x*P^3-5.675e-09*P^4-0.0004611*x^5+9.334e-07*x^4*P-1.221e-08*x^3*P^2-1.463e-09*x^2*P^3-4.929e-11*x*P^4+2.492e-12*P^5;
%Defining F and x vectors for the 6 actuators
F2 = zeros(length(P2),1); %6x1
x2 = zeros(length(P2),1); %6x1
% Transform P from bar to Kpa
P2 = 100*P2;

for i=1:length(P2)
% Obtaining the stroke
x2(i) = x_muscle2(i); 
% Obtaining the applied force
F2(i) = curve(x2(i),P2(i));
if F2(i)<0
    F2(i) = 0;
end
end
end

== matlab function walkingRobotRL3D/Walking Robot/DYNAMIC MODEL OF PAM FOR LEFT LEG/Dynamic Model Antagonisitic PAM1/Proportional Regulator (Muscles 1) ==
  data: V1 input; reg_type input; p1 output
% Author: Eduardo Reyero Ibáñez
% Descrition: In this file it will be implemented the required input for the PAM
function p1  = propReg(V1,reg_type)
%% Proportional pressure regulators VPPM
%Range of Voltage
minVoltage = 0;
maxVoltage = 7.98; % This voltage provide 8 bar of pressure with regulator type 1
p1 = zeros(1,1);
%Select regulartor type
%reg_type = 1; % This will be given by the call of the function
%Limit the voltage
for i=1:length(p1)
if V1(i) >= maxVoltage 
    V1(i) = maxVoltage;
end
end
if reg_type == 1
    f_prop = @(V) 0.99*V+0.1;
    for i=1:length(p1)
    p1(i) = f_prop(V1(i));
    end
elseif reg_type == 2
    f_prop = @(V) 0.594*V+0.06;
    for i=1:length(p1)
    p1(i) = f_prop(V1(i));
    end
else
    f_prop = @(V) 0.198*V+0.02;
    for i=1:length(p1)
    p1(i) = f_prop(V1(i));
    end
end

% figure
% fplot(p1)
% xlim([0 10])
% ylim([0 10])
end

== matlab function walkingRobotRL3D/Walking Robot/DYNAMIC MODEL OF PAM FOR LEFT LEG/Dynamic Model Antagonisitic PAM1/Proportional Regulator (Muscles 2) ==
  data: V1 input; reg_type input; p1 output
% Author: Eduardo Reyero Ibáñez
% Descrition: In this file it will be implemented the required input for the PAM
function p1  = propReg(V1,reg_type)
%% Proportional pressure regulators VPPM
%Range of Voltage
minVoltage = 0;
maxVoltage = 7.98; % This voltage provide 8 bar of pressure with regulator type 1
p1 = zeros(1,1);
%Select regulartor type
%reg_type = 1; % This will be given by the call of the function
%Limit the voltage
for i=1:length(p1)
if V1(i) >= maxVoltage 
    V1(i) = maxVoltage;
end
end
if reg_type == 1
    f_prop = @(V) 0.99*V+0.1;
    for i=1:length(p1)
    p1(i) = f_prop(V1(i));
    end
elseif reg_type == 2
    f_prop = @(V) 0.594*V+0.06;
    for i=1:length(p1)
    p1(i) = f_prop(V1(i));
    end
else
    f_prop = @(V) 0.198*V+0.02;
    for i=1:length(p1)
    p1(i) = f_prop(V1(i));
    end
end

% figure
% fplot(p1)
% xlim([0 10])
% ylim([0 10])
end

== matlab function walkingRobotRL3D/Walking Robot/DYNAMIC MODEL OF PAM FOR LEFT LEG/Dynamic Model Antagonisitic PAM1/Spring and damping model/S(P),D(P) ==
  data: P1 input; S1 output; P2 input; D1 output; S2 output; D2 output
function [S1,D1,S2,D2] = getSpringDampingCoeff(P1,P2)
tau = 0.6;
% Spring and damping coeff for muscle 1
if P1>=0 && P1<=1
    S1 = 400;
    D1 = tau*S1;
elseif P1>1 && P1<=2
    S1 = 500;
    D1 = tau*S1;
elseif P1>2 && P1<=3
    S1 = 1100;
    D1 = tau*S1;
elseif P1>3 && P1<=4
    S1 = 1500;
    D1 = tau*S1;
elseif P1>4 && P1<=5
    S1 = 2000;
    D1 = tau*S1;
elseif P1>5 && P1<=6
    S1 = 2900;
    D1 = tau*S1;
elseif P1>6 && P1<=7
    S1 = 3800;
    D1 = tau*S1;
elseif P1>7 && P1<=8.5
    S1 = 5000;
    D1 = tau*S1;
else %Never will enter here
    S1 = 800;
    D1 = tau*S1;  
end

% Spring and damping coeff for muscle 1
if P2>=0 && P2<=1
    S2 = 400;
    D2 = tau*S2;
elseif P2>1 && P2<=2
    S2 = 500;
    D2 = tau*S2;
elseif P2>2 && P2<=3
    S2 = 1100;
    D2 = tau*S2;
elseif P2>3 && P2<=4
    S2 = 1500;
    D2 = tau*S2;
elseif P2>4 && P2<=5
    S2 = 2000;
    D2 = tau*S2;
elseif P2>5 && P2<=6
    S2 = 2900;
    D2 = tau*S2;
elseif P2>6 && P2<=7
    S2 = 3800;
    D2 = tau*S2;
elseif P2>7 && P2<=8.5
    S2 = 5000;
    D2 = tau*S2;
else %Never will enter here
    S2 = 800;
    D2 = tau*S2;  
end

end

== matlab function walkingRobotRL3D/Walking Robot/DYNAMIC MODEL OF PAM FOR LEFT LEG/Dynamic Model Antagonisitic PAM2/F(x,P) mode (Muscles 1) ==
  data: P1 input; F1 output; x_muscle1 input
%Author: Eduardo Reyero Ibáñez
%Note: F(x) curves for different pressures are limited by recommended
%limitation of 20% in contraction percentage for the used PAM actuator
%(L = 260mm D=20mm)
function F1 = FxPmodel(P1,x_muscle1)
%Input: P comming from proporcional controller  is in bar. Its 6x1 vector
% x_muscle (in % contraction)
%Output:F according to P input and and x value of half of the maximun
%permissible stroke
%Importing 2 variable F(x,P) model
curve = @(x,P)  -0.002697-93.8*x+2.917*P+13.05*x^2-0.04264*x*P-0.001793*P^2-0.9395*x^3-0.001597*x^2*P-0.0001142*x*P^2+4.694e-06*P^3+0.03335*x^4+6.106e-06*x^3*P+2.699e-06*x^2*P^2+1.25e-07*x*P^3-5.675e-09*P^4-0.0004611*x^5+9.334e-07*x^4*P-1.221e-08*x^3*P^2-1.463e-09*x^2*P^3-4.929e-11*x*P^4+2.492e-12*P^5;
%Defining F and x vectors for the 6 actuators
F1 = zeros(length(P1),1); %6x1
x1 = zeros(length(P1),1); %6x1
% Transform P from bar to Kpa
P1 = 100*P1;

for i=1:length(P1)
% Obtaining the stroke
x1(i) = x_muscle1(i); 
% Obtaining the applied force
F1(i) = curve(x1(i),P1(i)); 
if F1(i)<0
    F1(i) = 0;
end
end
end

== matlab function walkingRobotRL3D/Walking Robot1/Dynamic model of antagonistic PAM actuators/Spring//Damping (Muscles 2)/Getxmax2/getMaxStroke1 ==
  data: P2 input; x_max2 output
%Author: Eduardo Reyero Ibáñez
%Description: Functions for obtaining the maximun stroke value of a given
%curve F(x). It is reached for the x value which makes F = 0
function x_max2 = getMaxStroke(P2)
x_range = (-3:0.01:29)'; %This range convers the %contraction for all the pressures from 0 to 8 bar
%load('StaticFxPmodel\fxpSurface.mat');
curve1 = @(x,P)  -0.002697-93.8*x+2.917*P+13.05*x^2-0.04264*x*P-0.001793*P^2-0.9395*x^3-0.001597*x^2*P-0.0001142*x*P^2+4.694e-06*P^3+0.03335*x^4+6.106e-06*x^3*P+2.699e-06*x^2*P^2+1.25e-07*x*P^3-5.675e-09*P^4-0.0004611*x^5+9.334e-07*x^4*P-1.221e-08*x^3*P^2-1.463e-09*x^2*P^3-4.929e-11*x*P^4+2.492e-12*P^5;
F_x = zeros(length(x_range),1);
for i=1:length(x_range)
    F_x(i) = curve1(x_range(i),P2);
    if F_x(i)<0
       %We have found the x axis cross
       x_max2 = x_range(i-1);
       break;
    else
        x_max2 = x_range(i); %Will never end here but need to avoid simulink error
    end
end

end

== matlab function walkingRobotRL3D/Walking Robot/DYNAMIC MODEL OF PAM FOR LEFT LEG/Dynamic Model Antagonisitic PAM2/F(x,P) mode (Muscles 1)1 ==
  data: P2 input; F2 output; x_muscle2 input
%Author: Eduardo Reyero Ibáñez
%Note: F(x) curves for different pressures are limited by recommended
%limitation of 20% in contraction percentage for the used PAM actuator
%(L = 260mm D=20mm)
function F2 = FxPmodel(P2,x_muscle2)
%Input: P comming from proporcional controller  is in bar. Its 6x1 vector
% x_muscle (in % contraction)
%Output:F according to P input and and x value of half of the maximun
%permissible stroke
%Importing 2 variable F(x,P) model
curve = @(x,P)  -0.002697-93.8*x+2.917*P+13.05*x^2-0.04264*x*P-0.001793*P^2-0.9395*x^3-0.001597*x^2*P-0.0001142*x*P^2+4.694e-06*P^3+0.03335*x^4+6.106e-06*x^3*P+2.699e-06*x^2*P^2+1.25e-07*x*P^3-5.675e-09*P^4-0.0004611*x^5+9.334e-07*x^4*P-1.221e-08*x^3*P^2-1.463e-09*x^2*P^3-4.929e-11*x*P^4+2.492e-12*P^5;
%Defining F and x vectors for the 6 actuators
F2 = zeros(length(P2),1); %6x1
x2 = zeros(length(P2),1); %6x1
% Transform P from bar to Kpa
P2 = 100*P2;

for i=1:length(P2)
% Obtaining the stroke
x2(i) = x_muscle2(i); 
% Obtaining the applied force
F2(i) = curve(x2(i),P2(i));
if F2(i)<0
    F2(i) = 0;
end
end
end
